simulink model "Logic_Final_Project_PRODUCT4_QUESTION37"  (R2025b)
settings: Solver=VariableStepAuto  StartTime=0.0  StopTime=100  RelTol=1e-3
libraries: simulink_extras x83
(part 2 of 2)

== system Logic_Final_Project_PRODUCT4_QUESTION37/Implemention 3/Machine-M6/D1 ==
  Q2! : Inport
  Q1 : Inport  Port=2
  Q1! : Inport  Port=3
  Q0! : Inport  Port=4
  Q0 : Inport  Port=5
  Enable : Inport  Port=6
  Logical Operator : Logic  AllPortsSameDT=off  OutDataTypeStr=boolean
  Logical Operator1 : Logic  Operator=NOT  AllPortsSameDT=off  OutDataTypeStr=boolean
  Logical Operator2 : Logic  AllPortsSameDT=off  OutDataTypeStr=boolean
  Logical Operator3 : Logic  Inputs=4  AllPortsSameDT=off  OutDataTypeStr=boolean
  Logical Operator4 : Logic  Operator=OR  Inputs=3  AllPortsSameDT=off  OutDataTypeStr=boolean
  D1 : Outport
  wires:
  Logical Operator4/1 -> D1/1
  Logical Operator/1 -> Logical Operator4/3
  Logical Operator2/1 -> Logical Operator4/2
  Logical Operator3/1 -> Logical Operator4/1
  Q0!/1 -> Logical Operator2/2
  Q2!/1 -> Logical Operator3/1
  Enable/1 -> Logical Operator1/1, Logical Operator3/4
  Q1/1 -> Logical Operator/1, Logical Operator2/1
  Q1!/1 -> Logical Operator3/3
  Logical Operator1/1 -> Logical Operator/2
  Q0/1 -> Logical Operator3/2

== system Logic_Final_Project_PRODUCT4_QUESTION37/Implemention 3/Machine-M6/D2  ==
  Q2 : Inport
  Q1 : Inport  Port=2
  Enable : Inport  Port=3
  Q0 : Inport  Port=4
  Q0! : Inport  Port=5
  Logical Operator : Logic  Operator=NOT  AllPortsSameDT=off  OutDataTypeStr=boolean
  Logical Operator1 : Logic  AllPortsSameDT=off  OutDataTypeStr=boolean
  Logical Operator2 : Logic  AllPortsSameDT=off  OutDataTypeStr=boolean
  Logical Operator3 : Logic  Inputs=3  AllPortsSameDT=off  OutDataTypeStr=boolean
  Logical Operator4 : Logic  Operator=OR  Inputs=3  AllPortsSameDT=off  OutDataTypeStr=boolean
  D2 : Outport
  wires:
  Logical Operator4/1 -> D2/1
  Q0!/1 -> Logical Operator2/2
  Enable/1 -> Logical Operator3/3, Logical Operator/1
  Logical Operator2/1 -> Logical Operator4/1
  Logical Operator1/1 -> Logical Operator4/2
  Logical Operator/1 -> Logical Operator1/2
  Logical Operator3/1 -> Logical Operator4/3
  Q1/1 -> Logical Operator3/1
  Q2/1 -> Logical Operator1/1, Logical Operator2/1
  Q0/1 -> Logical Operator3/2

== system Logic_Final_Project_PRODUCT4_QUESTION37/Implemention 3/Machine-M6/Machine_M6 ==
  ENBL : Inport
  CLK : Inport  Port=2
  D Flip-Flop 0 : simulink_extras/Flip Flops/D Flip-Flop
  D Flip-Flop1 : simulink_extras/Flip Flops/D Flip-Flop
  D Flip-Flop2 : simulink_extras/Flip Flops/D Flip-Flop
  Logical Operator : Logic  Operator=XOR  AllPortsSameDT=off  OutDataTypeStr=boolean
  Logical Operator1 : Logic  AllPortsSameDT=off  OutDataTypeStr=boolean
  Logical Operator2 : Logic  AllPortsSameDT=off  OutDataTypeStr=boolean
  Logical Operator3 : Logic  Operator=XOR  AllPortsSameDT=off  OutDataTypeStr=boolean
  Done : Outport
  wires:
  Logical Operator2/1 -> Done/1
  CLK/1 -> D Flip-Flop2/2, D Flip-Flop1/2, D Flip-Flop 0/2
  ENBL/1 -> D Flip-Flop1/3, D Flip-Flop2/3, D Flip-Flop 0/3
  Logical Operator3/1 -> D Flip-Flop2/1
  D Flip-Flop2/1 -> Logical Operator3/2, Logical Operator2/2
  Logical Operator1/1 -> Logical Operator3/1
  Logical Operator/1 -> D Flip-Flop1/1
  D Flip-Flop1/1 -> Logical Operator/2, Logical Operator1/2, Logical Operator2/1
  D Flip-Flop 0/1 -> Logical Operator/1, Logical Operator1/1
  D Flip-Flop 0/2 -> D Flip-Flop 0/1

== system Logic_Final_Project_PRODUCT4_QUESTION37/Implemention 3/Machine-M7/D0 ==
  Enable : Inport
  Q0! : Inport  Port=2
  Q0 : Inport  Port=3
  Logical Operator : Logic  AllPortsSameDT=off  OutDataTypeStr=boolean
  Logical Operator1 : Logic  Operator=NOT  AllPortsSameDT=off  OutDataTypeStr=boolean
  Logical Operator2 : Logic  Operator=OR  AllPortsSameDT=off  OutDataTypeStr=boolean
  Logical Operator3 : Logic  AllPortsSameDT=off  OutDataTypeStr=boolean
  D0 : Outport
  wires:
  Logical Operator1/1 -> Logical Operator/2
  Logical Operator/1 -> Logical Operator2/2
  Logical Operator2/1 -> D0/1
  Logical Operator3/1 -> Logical Operator2/1
  Enable/1 -> Logical Operator1/1, Logical Operator3/1
  Q0!/1 -> Logical Operator3/2
  Q0/1 -> Logical Operator/1

== system Logic_Final_Project_PRODUCT4_QUESTION37/Implemention 3/Machine-M7/D1 ==
  Q2! : Inport
  Q1 : Inport  Port=2
  Q1! : Inport  Port=3
  Q0! : Inport  Port=4
  Q0 : Inport  Port=5
  Enable : Inport  Port=6
  Logical Operator : Logic  AllPortsSameDT=off  OutDataTypeStr=boolean
  Logical Operator1 : Logic  Operator=NOT  AllPortsSameDT=off  OutDataTypeStr=boolean
  Logical Operator2 : Logic  AllPortsSameDT=off  OutDataTypeStr=boolean
  Logical Operator3 : Logic  Inputs=4  AllPortsSameDT=off  OutDataTypeStr=boolean
  Logical Operator4 : Logic  Operator=OR  Inputs=3  AllPortsSameDT=off  OutDataTypeStr=boolean
  D1 : Outport
  wires:
  Q0/1 -> Logical Operator3/2
  Logical Operator1/1 -> Logical Operator/2
  Q1!/1 -> Logical Operator3/3
  Q1/1 -> Logical Operator2/1, Logical Operator/1
  Enable/1 -> Logical Operator3/4, Logical Operator1/1
  Q2!/1 -> Logical Operator3/1
  Q0!/1 -> Logical Operator2/2
  Logical Operator3/1 -> Logical Operator4/1
  Logical Operator2/1 -> Logical Operator4/2
  Logical Operator/1 -> Logical Operator4/3
  Logical Operator4/1 -> D1/1

== system Logic_Final_Project_PRODUCT4_QUESTION37/Implemention 3/Machine-M7/D2  ==
  Q2 : Inport
  Q1 : Inport  Port=2
  Enable : Inport  Port=3
  Q0 : Inport  Port=4
  Q0! : Inport  Port=5
  Logical Operator : Logic  Operator=NOT  AllPortsSameDT=off  OutDataTypeStr=boolean
  Logical Operator1 : Logic  AllPortsSameDT=off  OutDataTypeStr=boolean
  Logical Operator2 : Logic  AllPortsSameDT=off  OutDataTypeStr=boolean
  Logical Operator3 : Logic  Inputs=3  AllPortsSameDT=off  OutDataTypeStr=boolean
  Logical Operator4 : Logic  Operator=OR  Inputs=3  AllPortsSameDT=off  OutDataTypeStr=boolean
  D2 : Outport
  wires:
  Q0/1 -> Logical Operator3/2
  Q2/1 -> Logical Operator2/1, Logical Operator1/1
  Q1/1 -> Logical Operator3/1
  Logical Operator3/1 -> Logical Operator4/3
  Logical Operator/1 -> Logical Operator1/2
  Logical Operator1/1 -> Logical Operator4/2
  Logical Operator2/1 -> Logical Operator4/1
  Enable/1 -> Logical Operator/1, Logical Operator3/3
  Q0!/1 -> Logical Operator2/2
  Logical Operator4/1 -> D2/1

== system Logic_Final_Project_PRODUCT4_QUESTION37/Implemention 3/Machine-M7/Machine_M7 ==
  ENBL : Inport
  CLK : Inport  Port=2
  D Flip-Flop 0 : simulink_extras/Flip Flops/D Flip-Flop
  D Flip-Flop1 : simulink_extras/Flip Flops/D Flip-Flop
  D Flip-Flop2 : simulink_extras/Flip Flops/D Flip-Flop
  Logical Operator : Logic  Operator=XOR  AllPortsSameDT=off  OutDataTypeStr=boolean
  Logical Operator1 : Logic  AllPortsSameDT=off  OutDataTypeStr=boolean
  Logical Operator3 : Logic  Operator=XOR  AllPortsSameDT=off  OutDataTypeStr=boolean
  Done : Outport
  wires:
  D Flip-Flop 0/2 -> D Flip-Flop 0/1
  D Flip-Flop 0/1 -> Logical Operator1/1, Logical Operator/1
  D Flip-Flop1/1 -> Done/1, Logical Operator1/2, Logical Operator/2
  Logical Operator/1 -> D Flip-Flop1/1
  Logical Operator1/1 -> Logical Operator3/1
  D Flip-Flop2/1 -> Logical Operator3/2
  Logical Operator3/1 -> D Flip-Flop2/1
  ENBL/1 -> D Flip-Flop 0/3, D Flip-Flop2/3, D Flip-Flop1/3
  CLK/1 -> D Flip-Flop 0/2, D Flip-Flop1/2, D Flip-Flop2/2

== stateflow chart Logic_Final_Project_PRODUCT4_QUESTION37/Implemention 1/Chart ==
  state IDLE
    en:
    Enable_M1=0;
    Enable_M3=0;
    Enable_M4=0;
    Enable_M6=0;
    Enable_M7=0;
  state M1_Active
    en:
    Enable_M1=1;
  state M3_Active
    en:
    Enable_M1=0;
    Enable_M3=1;
  state M4_Active
    en:
    Enable_M3=0;
    Enable_M4=1;
  state M6_Active
    en:
    Enable_M4=0;
    Enable_M6=1;
  state M7_Active
    en:
    Enable_M6=0;
    Enable_M7=1;
  (default) -> IDLE
  IDLE -> M1_Active : [Start == 1]
  M1_Active -> M3_Active : [Done_M1 == 1]
  M3_Active -> M4_Active : [Done_M3 == 1]
  M4_Active -> M6_Active : [Done_M4 == 1]
  M6_Active -> M7_Active : [Done_M6 == 1]
  M7_Active -> IDLE : [Done_M7 == 1]
  data: Start input; Done_M1 input; Done_M3 input; Done_M4 input; Done_M6 input; Done_M7 input; Enable_M1 output =0; Enable_M3 output =0; Enable_M4 output =0; Enable_M6 output =0; Enable_M7 output =0
